simulink model "ThreeWheeledVehicle"  (R2017b)
settings: Solver=VariableStepAuto  StartTime=0.0  StopTime=25  RelTol=1e-3
undefined symbols (not defined in the file): b_contact_RW, C_F_alpha, C_F_kappa, CM_phi, Cylinder, Dtheta0, epsilon, g, k_contact_RW, lengthRW, massRW, Parts_Lib, radiusRW, sigbuilder_block, sigma, X, xPla, Y, yPla, Z, zPla
libraries: nesl_utility x42, sm_lib x39, vrlib x21, simulink x3
(part 2 of 3)

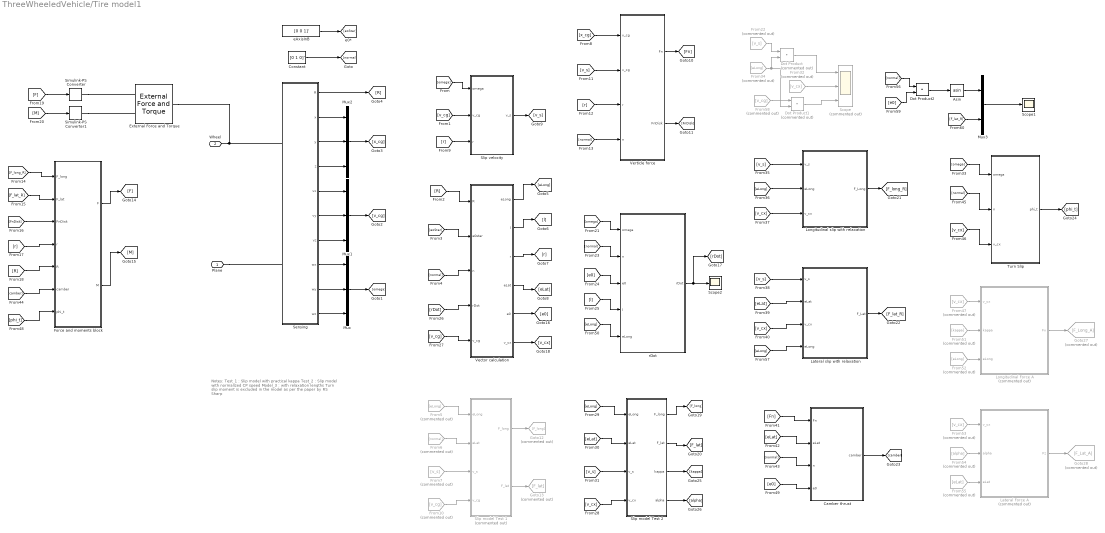
== system ThreeWheeledVehicle/Tire model1 ==
  note: Notes:
      | Test_1 : Slip model with practical kappa
      | Test_2 : Slip model with normalized CP speed
      | Model_3 : with relaxation lengths
      |
      | Turn slip moment is excluded in the model as per the
      | paper by RS Sharp
  Asin : Trigonometry  Operator=asin
  Camber thrust : Subsystem
  Constant : Constant  Value=[0 1 0]'
  Dot Product : DotProduct  Commented=on  InputSameDT=on  OutDataTypeStr=Inherit: Inherit via internal rule
  Dot Product1 : DotProduct  Commented=on  InputSameDT=on  OutDataTypeStr=Inherit: Inherit via internal rule
  Dot Product2 : DotProduct  InputSameDT=on  OutDataTypeStr=Inherit: Inherit via internal rule
  External Force and Torque : sm_lib/Forces and Torques/External Force and Torque  ForceResolutionFrame=AttachedFrame  EnableForceX=off  EnableForceY=off  EnableForceZ=off  EnableForce=on  TorqueResolutionFrame=AttachedFrame  EnableTorqueX=off  EnableTorqueY=off  EnableTorqueZ=off  EnableTorque=on
  Force and moments block : Subsystem
  From10 : From  Commented=on  GotoTag=v_cg
  From22 : From  Commented=on  GotoTag=v_s
  From32 : From  Commented=on  GotoTag=v_cx
  From34 : From  Commented=on  GotoTag=eLong
  From47 : From  Commented=on  GotoTag=v_cx
  From5 : From  Commented=on  GotoTag=eLong
  From51 : From  Commented=on  GotoTag=kappa
  From52 : From  Commented=on  GotoTag=eLong
  From53 : From  Commented=on  GotoTag=v_cx
  From54 : From  Commented=on  GotoTag=alpha
  From55 : From  Commented=on  GotoTag=eLat
  From58 : From  Commented=on  GotoTag=v_cg
  From6 : From  Commented=on  GotoTag=normal
  From7 : From  Commented=on  GotoTag=v_s
  Goto12 : Goto  Commented=on  GotoTag=F_long
  Goto13 : Goto  Commented=on  GotoTag=F_lat
  Goto27 : Goto  Commented=on  GotoTag=F_Long_A
  Goto28 : Goto  Commented=on  GotoTag=F_Lat_A
  Lateral Force A : Subsystem  Commented=on
  Lateral slip with relaxation : Subsystem
  Longitudinal Force A : Subsystem  Commented=on
  Longitudinal slip with relaxation : Subsystem
  Mux : Mux  Inputs=3
  Mux1 : Mux  Inputs=3
  Mux2 : Mux  Inputs=3
  Mux3 : Mux  Inputs=2
  Scope : Scope  Commented=on  NumInputPorts=3
  Scope1 : Scope
  Scope2 : Scope
  Sensing : Subsystem
  Simulink-PS Converter : nesl_utility/Simulink-PS Converter  PhysicalDomain=network_engine_domain  SubClassName=ps_input  LeftPortType=input  RightPortType=output  PseudoPeriodic=off  Frequencies=[]  NoiseDistribution=none  NoiseParameters=[]  Unit=N  AffineConversion=off  FilteringAndDerivatives=provide  SimscapeFilterOrder=1  InputFilterTimeConstant=0.001  UdotUserProvided=0
  Simulink-PS Converter1 : nesl_utility/Simulink-PS Converter  PhysicalDomain=network_engine_domain  SubClassName=ps_input  LeftPortType=input  RightPortType=output  PseudoPeriodic=off  Frequencies=[]  NoiseDistribution=none  NoiseParameters=[]  Unit=N*m  AffineConversion=off  FilteringAndDerivatives=provide  SimscapeFilterOrder=1  InputFilterTimeConstant=0.001  UdotUserProvided=0
  Slip model Test 1 : Subsystem  Commented=on
  Slip model Test 2 : Subsystem
  Slip velocity : Subsystem
  Turn Slip : Subsystem
  Vector calculation : Subsystem
  Verticle force : Subsystem
  eAxisInB : Constant  Value=[0 0 1]'
  rDot : Subsystem
  Plane : PMIOPort  Port=1  Side=Left
  Wheel : PMIOPort  Port=2  Side=Right
  wires:
  eAxisInB/1 -> [eoStar]
  Constant/1 -> [normal]
  Sensing/8(wx) -> Mux/1
  Sensing/9(wy) -> Mux/2
  Sensing/10(wz) -> Mux/3
  Mux/1 -> [omega]
  [omega] -> Slip velocity/1(omega)
  Sensing/5(vx) -> Mux1/1
  Sensing/6(vy) -> Mux1/2
  Sensing/7(vz) -> Mux1/3
  Mux1/1 -> [v_cg]
  [v_cg] -> Slip velocity/2(v_cg)
  Sensing/2(x) -> Mux2/1
  Sensing/3(y) -> Mux2/2
  Sensing/4(z) -> Mux2/3
  Mux2/1 -> [x_cg]
  Sensing/1(R) -> [R]
  [R] -> Vector calculation/1(R)
  [eoStar] -> Vector calculation/2(e0star)
  [normal] -> Vector calculation/3(n)
  From5/1 -> Slip model Test 1/1(eLong)
  From6/1 -> Slip model Test 1/2(eLat)
  Vector calculation/1(eLong) -> [eLong]
  Vector calculation/2(l) -> [l]
  Vector calculation/3(r) -> [r]
  Vector calculation/4(eLat) -> [eLat]
  [r] -> Slip velocity/3(r)
  Slip velocity/1(v_s) -> [v_s]
  From7/1 -> Slip model Test 1/3(v_s)
  From10/1 -> Slip model Test 1/4(v_cg)
  [x_cg] -> Verticle force/1(x_cg)
  [v_s] -> Verticle force/2(v_cg)
  [r] -> Verticle force/3(r)
  [normal] -> Verticle force/4(n)
  Verticle force/1(Fn) -> [Fn]
  Verticle force/2(FnDisk) -> [FnDisk]
  Slip model Test 1/1(F_long) -> Goto12/1
  Slip model Test 1/2(F_lat) -> Goto13/1
  [r] -> Force and moments block/4(r)
  [R] -> Force and moments block/5(R)
  [F] -> Simulink-PS Converter/1
  [M] -> Simulink-PS Converter1/1
  Vector calculation/5(e0) -> [e0]
  [v_cg] -> Vector calculation/5(v_cg)
  Vector calculation/6(v_cx) -> [v_cx]
  Slip model Test 2/1(F_long) -> [F_long]
  [v_s] -> Slip model Test 2/3(v_s)
  [eLat] -> Slip model Test 2/2(eLat)
  [eLong] -> Slip model Test 2/1(eLong)
  Slip model Test 2/2(F_lat) -> [F_lat]
  [v_cx] -> Slip model Test 2/4(v_cx)
  From22/1 -> Dot Product/1
  From34/1 -> Dot Product1/2, Dot Product/2
  Dot Product/1 -> Scope/1
  [v_s] -> Longitudinal slip with relaxation/1(v_s)
  [eLong] -> Longitudinal slip with relaxation/2(eLong)
  [v_cx] -> Longitudinal slip with relaxation/3(v_cx)
  Longitudinal slip with relaxation/1(F_Long) -> [F_long_R]
  [eLat] -> Lateral slip with relaxation/2(eLat)
  Lateral slip with relaxation/1(F_Lat) -> [F_lat_R]
  [v_cx] -> Lateral slip with relaxation/3(v_cx)
  [v_s] -> Lateral slip with relaxation/1(v_s)
  [Fn] -> Camber thrust/1(Fn)
  [eLat] -> Camber thrust/2(eLat)
  [normal] -> Camber thrust/3(n)
  Camber thrust/1(camber) -> [camber]
  [e0] -> Camber thrust/4(e0)
  Force and moments block/1(F) -> [F]
  Force and moments block/2(M) -> [M]
  [eLong] -> Lateral slip with relaxation/4(eLong)
  From32/1 -> Scope/2
  From58/1 -> Dot Product1/1
  Dot Product1/1 -> Scope/3
  [omega] -> rDot/1(omega)
  [normal] -> rDot/2(n)
  [e0] -> rDot/3(e0)
  [l] -> rDot/4(l)
  [eLong] -> rDot/5(eLong)
  rDot/1(rDot) -> [rDot], Scope2/1
  [rDot] -> Vector calculation/4(rDot)
  Slip model Test 2/3(kappa) -> [kappa]
  [omega] -> Turn Slip/1(omega)
  [normal] -> Turn Slip/2(n)
  [v_cx] -> Turn Slip/3(v_cx)
  Turn Slip/1(phi_t) -> [phi_t]
  From47/1 -> Longitudinal Force A/1(v_cx)
  Slip model Test 2/4(alpha) -> [alpha]
  From51/1 -> Longitudinal Force A/2(kappa)
  From52/1 -> Longitudinal Force A/3(eLong)
  Longitudinal Force A/1(Fx) -> Goto27/1
  From53/1 -> Lateral Force A/1(v_cx)
  From54/1 -> Lateral Force A/2(alpha)
  From55/1 -> Lateral Force A/3(eLat)
  Lateral Force A/1(Fz) -> Goto28/1
  [normal] -> Dot Product2/1
  [e0] -> Dot Product2/2
  Dot Product2/1 -> Asin/1
  Asin/1 -> Mux3/1
  [F_lat_R] -> Mux3/2
  Mux3/1 -> Scope1/1
  [FnDisk] -> Force and moments block/3(FnDisk)
  [F_long_R] -> Force and moments block/1(F_long)
  [F_lat_R] -> Force and moments block/2(F_lat)
  [camber] -> Force and moments block/6(camber)
  [phi_t] -> Force and moments block/7(phi_t)
  connections:
  Plane/RConn1 -- Sensing/LConn2
  Wheel/RConn1 -- External Force and Torque/RConn1 -- Sensing/LConn1
  Simulink-PS Converter/RConn1 -- External Force and Torque/LConn1
  Simulink-PS Converter1/RConn1 -- External Force and Torque/LConn2

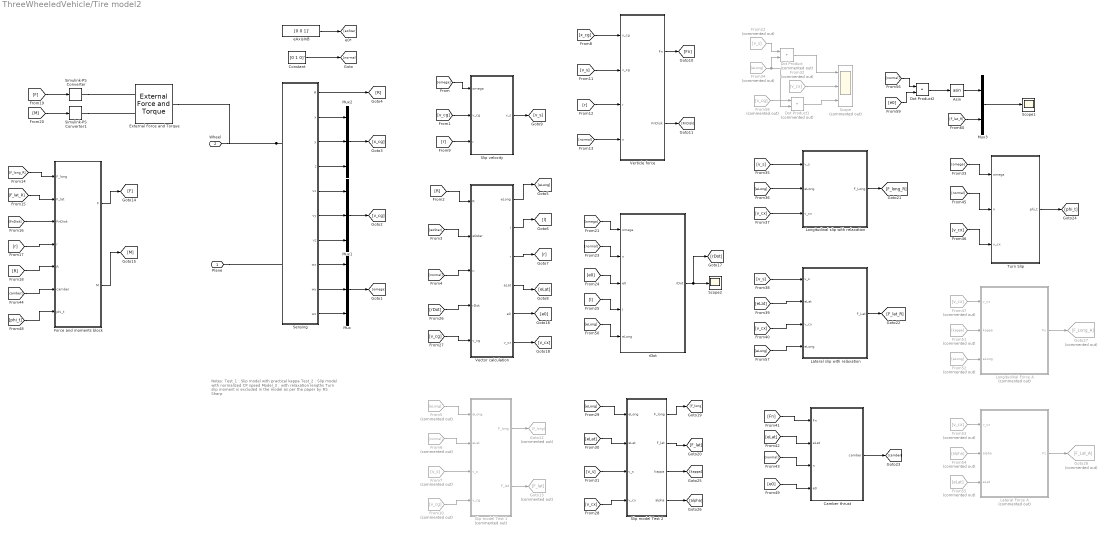
== system ThreeWheeledVehicle/Tire model2 ==
  note: Notes:
      | Test_1 : Slip model with practical kappa
      | Test_2 : Slip model with normalized CP speed
      | Model_3 : with relaxation lengths
      |
      | Turn slip moment is excluded in the model as per the
      | paper by RS Sharp
  Asin : Trigonometry  Operator=asin
  Camber thrust : Subsystem
  Constant : Constant  Value=[0 1 0]'
  Dot Product : DotProduct  Commented=on  InputSameDT=on  OutDataTypeStr=Inherit: Inherit via internal rule
  Dot Product1 : DotProduct  Commented=on  InputSameDT=on  OutDataTypeStr=Inherit: Inherit via internal rule
  Dot Product2 : DotProduct  InputSameDT=on  OutDataTypeStr=Inherit: Inherit via internal rule
  External Force and Torque : sm_lib/Forces and Torques/External Force and Torque  ForceResolutionFrame=AttachedFrame  EnableForceX=off  EnableForceY=off  EnableForceZ=off  EnableForce=on  TorqueResolutionFrame=AttachedFrame  EnableTorqueX=off  EnableTorqueY=off  EnableTorqueZ=off  EnableTorque=on
  Force and moments block : Subsystem
  From10 : From  Commented=on  GotoTag=v_cg
  From22 : From  Commented=on  GotoTag=v_s
  From32 : From  Commented=on  GotoTag=v_cx
  From34 : From  Commented=on  GotoTag=eLong
  From47 : From  Commented=on  GotoTag=v_cx
  From5 : From  Commented=on  GotoTag=eLong
  From51 : From  Commented=on  GotoTag=kappa
  From52 : From  Commented=on  GotoTag=eLong
  From53 : From  Commented=on  GotoTag=v_cx
  From54 : From  Commented=on  GotoTag=alpha
  From55 : From  Commented=on  GotoTag=eLat
  From58 : From  Commented=on  GotoTag=v_cg
  From6 : From  Commented=on  GotoTag=normal
  From7 : From  Commented=on  GotoTag=v_s
  Goto12 : Goto  Commented=on  GotoTag=F_long
  Goto13 : Goto  Commented=on  GotoTag=F_lat
  Goto27 : Goto  Commented=on  GotoTag=F_Long_A
  Goto28 : Goto  Commented=on  GotoTag=F_Lat_A
  Lateral Force A : Subsystem  Commented=on
  Lateral slip with relaxation : Subsystem
  Longitudinal Force A : Subsystem  Commented=on
  Longitudinal slip with relaxation : Subsystem
  Mux : Mux  Inputs=3
  Mux1 : Mux  Inputs=3
  Mux2 : Mux  Inputs=3
  Mux3 : Mux  Inputs=2
  Scope : Scope  Commented=on  NumInputPorts=3
  Scope1 : Scope
  Scope2 : Scope
  Sensing : Subsystem
  Simulink-PS Converter : nesl_utility/Simulink-PS Converter  PhysicalDomain=network_engine_domain  SubClassName=ps_input  LeftPortType=input  RightPortType=output  PseudoPeriodic=off  Frequencies=[]  NoiseDistribution=none  NoiseParameters=[]  Unit=N  AffineConversion=off  FilteringAndDerivatives=provide  SimscapeFilterOrder=1  InputFilterTimeConstant=0.001  UdotUserProvided=0
  Simulink-PS Converter1 : nesl_utility/Simulink-PS Converter  PhysicalDomain=network_engine_domain  SubClassName=ps_input  LeftPortType=input  RightPortType=output  PseudoPeriodic=off  Frequencies=[]  NoiseDistribution=none  NoiseParameters=[]  Unit=N*m  AffineConversion=off  FilteringAndDerivatives=provide  SimscapeFilterOrder=1  InputFilterTimeConstant=0.001  UdotUserProvided=0
  Slip model Test 1 : Subsystem  Commented=on
  Slip model Test 2 : Subsystem
  Slip velocity : Subsystem
  Turn Slip : Subsystem
  Vector calculation : Subsystem
  Verticle force : Subsystem
  eAxisInB : Constant  Value=[0 0 1]'
  rDot : Subsystem
  Plane : PMIOPort  Port=1  Side=Left
  Wheel : PMIOPort  Port=2  Side=Right
  wires:
  [camber] -> Force and moments block/6(camber)
  [F_lat_R] -> Force and moments block/2(F_lat)
  [F_long_R] -> Force and moments block/1(F_long)
  [FnDisk] -> Force and moments block/3(FnDisk)
  Mux3/1 -> Scope1/1
  [F_lat_R] -> Mux3/2
  Asin/1 -> Mux3/1
  Dot Product2/1 -> Asin/1
  [e0] -> Dot Product2/2
  [normal] -> Dot Product2/1
  Lateral Force A/1(Fz) -> Goto28/1
  From55/1 -> Lateral Force A/3(eLat)
  From54/1 -> Lateral Force A/2(alpha)
  From53/1 -> Lateral Force A/1(v_cx)
  Longitudinal Force A/1(Fx) -> Goto27/1
  From52/1 -> Longitudinal Force A/3(eLong)
  From51/1 -> Longitudinal Force A/2(kappa)
  Slip model Test 2/4(alpha) -> [alpha]
  From47/1 -> Longitudinal Force A/1(v_cx)
  Turn Slip/1(phi_t) -> [phi_t]
  [v_cx] -> Turn Slip/3(v_cx)
  [normal] -> Turn Slip/2(n)
  [omega] -> Turn Slip/1(omega)
  Slip model Test 2/3(kappa) -> [kappa]
  [rDot] -> Vector calculation/4(rDot)
  rDot/1(rDot) -> Scope2/1, [rDot]
  [eLong] -> rDot/5(eLong)
  [l] -> rDot/4(l)
  [e0] -> rDot/3(e0)
  [normal] -> rDot/2(n)
  [omega] -> rDot/1(omega)
  Dot Product1/1 -> Scope/3
  From58/1 -> Dot Product1/1
  From32/1 -> Scope/2
  [eLong] -> Lateral slip with relaxation/4(eLong)
  Force and moments block/2(M) -> [M]
  Force and moments block/1(F) -> [F]
  [e0] -> Camber thrust/4(e0)
  Camber thrust/1(camber) -> [camber]
  [normal] -> Camber thrust/3(n)
  [eLat] -> Camber thrust/2(eLat)
  [Fn] -> Camber thrust/1(Fn)
  [v_s] -> Lateral slip with relaxation/1(v_s)
  [v_cx] -> Lateral slip with relaxation/3(v_cx)
  Lateral slip with relaxation/1(F_Lat) -> [F_lat_R]
  [eLat] -> Lateral slip with relaxation/2(eLat)
  Longitudinal slip with relaxation/1(F_Long) -> [F_long_R]
  [v_cx] -> Longitudinal slip with relaxation/3(v_cx)
  [eLong] -> Longitudinal slip with relaxation/2(eLong)
  [v_s] -> Longitudinal slip with relaxation/1(v_s)
  Dot Product/1 -> Scope/1
  From34/1 -> Dot Product/2, Dot Product1/2
  From22/1 -> Dot Product/1
  [v_cx] -> Slip model Test 2/4(v_cx)
  Slip model Test 2/2(F_lat) -> [F_lat]
  [eLong] -> Slip model Test 2/1(eLong)
  [eLat] -> Slip model Test 2/2(eLat)
  [v_s] -> Slip model Test 2/3(v_s)
  Slip model Test 2/1(F_long) -> [F_long]
  Vector calculation/6(v_cx) -> [v_cx]
  [v_cg] -> Vector calculation/5(v_cg)
  Vector calculation/5(e0) -> [e0]
  [M] -> Simulink-PS Converter1/1
  [F] -> Simulink-PS Converter/1
  [R] -> Force and moments block/5(R)
  [r] -> Force and moments block/4(r)
  Slip model Test 1/2(F_lat) -> Goto13/1
  Slip model Test 1/1(F_long) -> Goto12/1
  Verticle force/2(FnDisk) -> [FnDisk]
  Verticle force/1(Fn) -> [Fn]
  [normal] -> Verticle force/4(n)
  [r] -> Verticle force/3(r)
  [v_s] -> Verticle force/2(v_cg)
  [x_cg] -> Verticle force/1(x_cg)
  From10/1 -> Slip model Test 1/4(v_cg)
  From7/1 -> Slip model Test 1/3(v_s)
  Slip velocity/1(v_s) -> [v_s]
  [r] -> Slip velocity/3(r)
  Vector calculation/4(eLat) -> [eLat]
  Vector calculation/3(r) -> [r]
  Vector calculation/2(l) -> [l]
  Vector calculation/1(eLong) -> [eLong]
  From6/1 -> Slip model Test 1/2(eLat)
  From5/1 -> Slip model Test 1/1(eLong)
  [normal] -> Vector calculation/3(n)
  [eoStar] -> Vector calculation/2(e0star)
  [R] -> Vector calculation/1(R)
  Sensing/1(R) -> [R]
  Mux2/1 -> [x_cg]
  Sensing/4(z) -> Mux2/3
  Sensing/3(y) -> Mux2/2
  Sensing/2(x) -> Mux2/1
  [v_cg] -> Slip velocity/2(v_cg)
  Mux1/1 -> [v_cg]
  Sensing/7(vz) -> Mux1/3
  Sensing/6(vy) -> Mux1/2
  Sensing/5(vx) -> Mux1/1
  [omega] -> Slip velocity/1(omega)
  Mux/1 -> [omega]
  Sensing/10(wz) -> Mux/3
  Sensing/9(wy) -> Mux/2
  Sensing/8(wx) -> Mux/1
  Constant/1 -> [normal]
  eAxisInB/1 -> [eoStar]
  [phi_t] -> Force and moments block/7(phi_t)
  connections:
  Simulink-PS Converter1/RConn1 -- External Force and Torque/LConn2
  Simulink-PS Converter/RConn1 -- External Force and Torque/LConn1
  Sensing/LConn1 -- External Force and Torque/RConn1 -- Wheel/RConn1
  Plane/RConn1 -- Sensing/LConn2

== system ThreeWheeledVehicle/Wheel_Front ==
  Cylinder : sm_lib/Body Elements/Solid  InertiaType=Custom  Mass=massRW  MassUnits=kg  CenterOfMass=[0 0 0]  CenterOfMassUnits=m  MomentsOfInertia=momentInertiaRW  MomentsOfInertiaUnits=kg*m^2  ProductsOfInertia=[0 0 0]  ProductsOfInertiaUnits=kg*m^2  DensityBased=on  Density=cyl_density  DensityUnits=kg/(m^3)  DoExposeReferenceFrame=on  SerializedFrames=<Frames/>  GraphicType=FromGeometry  MarkerShape=Sphere  MarkerSize=10  MarkerSizeUnits=m  GraphicVisPropType=SimpleVisualProperties  GraphicDiffuseColor=[0.0 0.5 0.7]  GraphicSpecularColor=[0.5 0.5 0.5 1.0]  GraphicAmbientColor=[0.15 0.15 0.15 1.0]  GraphicEmissiveColor=[0.0 0.0 0.0 1.0]  GraphicShininess=75  GraphicOpacity=cyl_opacity  GeometryShape=Cylinder  RectangleSize=[1 1]  RectangleSizeUnits=m  BrickDimensions=[1 1 1]  BrickDimensionUnits=m  CylinderRadius=cyl_radius  CylinderRadiusUnits=m  CylinderLength=cyl_length  CylinderLengthUnits=m  SphereRadius=1  SphereRadiusUnits=m  EllipsoidRadii=[1 1 1]  EllipsoidRadiiUnits=m  ExtrusionCrossSection=[1 1; -1 1; -1 -1; 1 -1]  ExtrusionCrossSectionUnits=m  ExtrusionLength=1  ExtrusionLengthUnits=m  PolygonNumSides=3  PolygonOuterRadius=1  PolygonOuterRadiusUnits=m  ExtGeomFileType=STL  ExtGeomFileUnits=m  RevolutionCrossSection=[1 1; 1 -1; 2 -1; 2 1]  RevolutionCrossSectionUnits=m  RevolutionExtent=Full  RevolutionAngle=180  RevolutionAngleUnits=deg
  Transform Vis2 : sm_lib/Frames and Transforms/Rigid Transform  TranslationMethod=None  TranslationStandardOffset=0  TranslationLengthUnit=m  TranslationStandardAxis=+Z  TranslationCartesianOffset=[0 0 0]  TranslationROffset=0  TranslationROffsetUnits=m  TranslationZOffset=0  TranslationZOffsetUnits=m  TranslationThetaOffset=0  TranslationThetaOffsetUnits=deg  RotationMethod=StandardAxis  RotationAngleUnits=deg  RotationStandardAxis=+Y  RotationAngle=180  RotationArbitraryAxis=[0 0 1]  FollAlignAxisA=+X  BaseAlignAxisA=+Y  FollAlignAxisB=+Y  BaseAlignAxisB=+Z  RotationSequenceAxes=FollowerAxes  RotationSequence=XYX  RotationSequenceAngles=[0 0 0]  RotationSequenceAnglesUnits=deg  RotationMatrix=[1 0 0; 0 1 0; 0 0 1]
  Vis1 : sm_lib/Body Elements/Solid  InertiaType=CalculateFromGeometry  Mass=1  MassUnits=kg  CenterOfMass=[0 0 0]  CenterOfMassUnits=m  MomentsOfInertia=[1 1 1]  MomentsOfInertiaUnits=kg*m^2  ProductsOfInertia=[0 0 0]  ProductsOfInertiaUnits=kg*m^2  DensityBased=on  Density=1e-3  DensityUnits=kg/(m^3)  DoExposeReferenceFrame=on  SerializedFrames=<Frames/>  GraphicType=FromGeometry  MarkerShape=Sphere  MarkerSize=10  MarkerSizeUnits=m  GraphicVisPropType=SimpleVisualProperties  GraphicDiffuseColor=[0.4 0.0 0.4]  GraphicSpecularColor=[0.5 0.5 0.5 1.0]  GraphicAmbientColor=[0.15 0.15 0.15 1.0]  GraphicEmissiveColor=[0.0 0.0 0.0 1.0]  GraphicShininess=75  GraphicOpacity=mark_opacity  GeometryShape=GeneralSolidOfRevolution  RectangleSize=[1 1]  RectangleSizeUnits=m  BrickDimensions=[1 1 1]  BrickDimensionUnits=m  CylinderRadius=0.1  CylinderRadiusUnits=m  CylinderLength=0.01  CylinderLengthUnits=m  SphereRadius=1  SphereRadiusUnits=m  EllipsoidRadii=[1 1 1]  EllipsoidRadiiUnits=m  ExtrusionCrossSection=[1 1; -1 1; -1 -1; 1 -1]  ExtrusionCrossSectionUnits=m  ExtrusionLength=1  ExtrusionLengthUnits=m  PolygonNumSides=3  PolygonOuterRadius=1  PolygonOuterRadiusUnits=m  ExtGeomFileType=STL  ExtGeomFileUnits=m  RevolutionCrossSection=[cyl_radius*mark_radius(1) cyl_length/2*mark_len_factor; cyl_radius*mark_radius(2) cyl_length/2*mark_len_factor; cyl_radius*mark_radius(2) -cyl_length/2*mark_len_factor; cyl_radius*mark_radius(1) -cyl_length/2*mark_len_factor]  RevolutionCrossSectionUnits=m  RevolutionExtent=Custom  RevolutionAngle=mark_angle  RevolutionAngleUnits=deg
  Vis2 : sm_lib/Body Elements/Solid  InertiaType=CalculateFromGeometry  Mass=1  MassUnits=kg  CenterOfMass=[0 0 0]  CenterOfMassUnits=m  MomentsOfInertia=[1 1 1]  MomentsOfInertiaUnits=kg*m^2  ProductsOfInertia=[0 0 0]  ProductsOfInertiaUnits=kg*m^2  DensityBased=on  Density=1e-3  DensityUnits=kg/(m^3)  DoExposeReferenceFrame=on  SerializedFrames=<Frames/>  GraphicType=FromGeometry  MarkerShape=Sphere  MarkerSize=10  MarkerSizeUnits=m  GraphicVisPropType=SimpleVisualProperties  GraphicDiffuseColor=[0.4 0.0 0.4]  GraphicSpecularColor=[0.5 0.5 0.5 1.0]  GraphicAmbientColor=[0.15 0.15 0.15 1.0]  GraphicEmissiveColor=[0.0 0.0 0.0 1.0]  GraphicShininess=75  GraphicOpacity=mark_opacity  GeometryShape=GeneralSolidOfRevolution  RectangleSize=[1 1]  RectangleSizeUnits=m  BrickDimensions=[1 1 1]  BrickDimensionUnits=m  CylinderRadius=0.1  CylinderRadiusUnits=m  CylinderLength=0.01  CylinderLengthUnits=m  SphereRadius=1  SphereRadiusUnits=m  EllipsoidRadii=[1 1 1]  EllipsoidRadiiUnits=m  ExtrusionCrossSection=[1 1; -1 1; -1 -1; 1 -1]  ExtrusionCrossSectionUnits=m  ExtrusionLength=1  ExtrusionLengthUnits=m  PolygonNumSides=3  PolygonOuterRadius=1  PolygonOuterRadiusUnits=m  ExtGeomFileType=STL  ExtGeomFileUnits=m  RevolutionCrossSection=[cyl_radius*mark_radius(1) cyl_length/2*mark_len_factor; cyl_radius*mark_radius(2) cyl_length/2*mark_len_factor; cyl_radius*mark_radius(2) -cyl_length/2*mark_len_factor; cyl_radius*mark_radius(1) -cyl_length/2*mark_len_factor]  RevolutionCrossSectionUnits=m  RevolutionExtent=Custom  RevolutionAngle=mark_angle  RevolutionAngleUnits=deg
  R : PMIOPort  Port=1  Side=Left
  connections:
  R/RConn1 -- Cylinder/RConn1 -- Transform Vis2/LConn1 -- Vis1/RConn1
  Vis2/RConn1 -- Transform Vis2/RConn1

== system ThreeWheeledVehicle/Wheel_RW_L ==
  Cylinder : sm_lib/Body Elements/Solid  InertiaType=Custom  Mass=massRW  MassUnits=kg  CenterOfMass=[0 0 0]  CenterOfMassUnits=m  MomentsOfInertia=momentInertiaRW  MomentsOfInertiaUnits=kg*m^2  ProductsOfInertia=[0 0 0]  ProductsOfInertiaUnits=kg*m^2  DensityBased=on  Density=cyl_density  DensityUnits=kg/(m^3)  DoExposeReferenceFrame=on  SerializedFrames=<Frames/>  GraphicType=FromGeometry  MarkerShape=Sphere  MarkerSize=10  MarkerSizeUnits=m  GraphicVisPropType=SimpleVisualProperties  GraphicDiffuseColor=[0.0 0.5 0.7]  GraphicSpecularColor=[0.5 0.5 0.5 1.0]  GraphicAmbientColor=[0.15 0.15 0.15 1.0]  GraphicEmissiveColor=[0.0 0.0 0.0 1.0]  GraphicShininess=75  GraphicOpacity=cyl_opacity  GeometryShape=Cylinder  RectangleSize=[1 1]  RectangleSizeUnits=m  BrickDimensions=[1 1 1]  BrickDimensionUnits=m  CylinderRadius=cyl_radius  CylinderRadiusUnits=m  CylinderLength=cyl_length  CylinderLengthUnits=m  SphereRadius=1  SphereRadiusUnits=m  EllipsoidRadii=[1 1 1]  EllipsoidRadiiUnits=m  ExtrusionCrossSection=[1 1; -1 1; -1 -1; 1 -1]  ExtrusionCrossSectionUnits=m  ExtrusionLength=1  ExtrusionLengthUnits=m  PolygonNumSides=3  PolygonOuterRadius=1  PolygonOuterRadiusUnits=m  ExtGeomFileType=STL  ExtGeomFileUnits=m  RevolutionCrossSection=[1 1; 1 -1; 2 -1; 2 1]  RevolutionCrossSectionUnits=m  RevolutionExtent=Full  RevolutionAngle=180  RevolutionAngleUnits=deg
  Transform Vis2 : sm_lib/Frames and Transforms/Rigid Transform  TranslationMethod=None  TranslationStandardOffset=0  TranslationLengthUnit=m  TranslationStandardAxis=+Z  TranslationCartesianOffset=[0 0 0]  TranslationROffset=0  TranslationROffsetUnits=m  TranslationZOffset=0  TranslationZOffsetUnits=m  TranslationThetaOffset=0  TranslationThetaOffsetUnits=deg  RotationMethod=StandardAxis  RotationAngleUnits=deg  RotationStandardAxis=+Y  RotationAngle=180  RotationArbitraryAxis=[0 0 1]  FollAlignAxisA=+X  BaseAlignAxisA=+Y  FollAlignAxisB=+Y  BaseAlignAxisB=+Z  RotationSequenceAxes=FollowerAxes  RotationSequence=XYX  RotationSequenceAngles=[0 0 0]  RotationSequenceAnglesUnits=deg  RotationMatrix=[1 0 0; 0 1 0; 0 0 1]
  Vis1 : sm_lib/Body Elements/Solid  InertiaType=CalculateFromGeometry  Mass=1  MassUnits=kg  CenterOfMass=[0 0 0]  CenterOfMassUnits=m  MomentsOfInertia=[1 1 1]  MomentsOfInertiaUnits=kg*m^2  ProductsOfInertia=[0 0 0]  ProductsOfInertiaUnits=kg*m^2  DensityBased=on  Density=1e-3  DensityUnits=kg/(m^3)  DoExposeReferenceFrame=on  SerializedFrames=<Frames/>  GraphicType=FromGeometry  MarkerShape=Sphere  MarkerSize=10  MarkerSizeUnits=m  GraphicVisPropType=SimpleVisualProperties  GraphicDiffuseColor=[0.4 0.0 0.4]  GraphicSpecularColor=[0.5 0.5 0.5 1.0]  GraphicAmbientColor=[0.15 0.15 0.15 1.0]  GraphicEmissiveColor=[0.0 0.0 0.0 1.0]  GraphicShininess=75  GraphicOpacity=mark_opacity  GeometryShape=GeneralSolidOfRevolution  RectangleSize=[1 1]  RectangleSizeUnits=m  BrickDimensions=[1 1 1]  BrickDimensionUnits=m  CylinderRadius=0.1  CylinderRadiusUnits=m  CylinderLength=0.01  CylinderLengthUnits=m  SphereRadius=1  SphereRadiusUnits=m  EllipsoidRadii=[1 1 1]  EllipsoidRadiiUnits=m  ExtrusionCrossSection=[1 1; -1 1; -1 -1; 1 -1]  ExtrusionCrossSectionUnits=m  ExtrusionLength=1  ExtrusionLengthUnits=m  PolygonNumSides=3  PolygonOuterRadius=1  PolygonOuterRadiusUnits=m  ExtGeomFileType=STL  ExtGeomFileUnits=m  RevolutionCrossSection=[cyl_radius*mark_radius(1) cyl_length/2*mark_len_factor; cyl_radius*mark_radius(2) cyl_length/2*mark_len_factor; cyl_radius*mark_radius(2) -cyl_length/2*mark_len_factor; cyl_radius*mark_radius(1) -cyl_length/2*mark_len_factor]  RevolutionCrossSectionUnits=m  RevolutionExtent=Custom  RevolutionAngle=mark_angle  RevolutionAngleUnits=deg
  Vis2 : sm_lib/Body Elements/Solid  InertiaType=CalculateFromGeometry  Mass=1  MassUnits=kg  CenterOfMass=[0 0 0]  CenterOfMassUnits=m  MomentsOfInertia=[1 1 1]  MomentsOfInertiaUnits=kg*m^2  ProductsOfInertia=[0 0 0]  ProductsOfInertiaUnits=kg*m^2  DensityBased=on  Density=1e-3  DensityUnits=kg/(m^3)  DoExposeReferenceFrame=on  SerializedFrames=<Frames/>  GraphicType=FromGeometry  MarkerShape=Sphere  MarkerSize=10  MarkerSizeUnits=m  GraphicVisPropType=SimpleVisualProperties  GraphicDiffuseColor=[0.4 0.0 0.4]  GraphicSpecularColor=[0.5 0.5 0.5 1.0]  GraphicAmbientColor=[0.15 0.15 0.15 1.0]  GraphicEmissiveColor=[0.0 0.0 0.0 1.0]  GraphicShininess=75  GraphicOpacity=mark_opacity  GeometryShape=GeneralSolidOfRevolution  RectangleSize=[1 1]  RectangleSizeUnits=m  BrickDimensions=[1 1 1]  BrickDimensionUnits=m  CylinderRadius=0.1  CylinderRadiusUnits=m  CylinderLength=0.01  CylinderLengthUnits=m  SphereRadius=1  SphereRadiusUnits=m  EllipsoidRadii=[1 1 1]  EllipsoidRadiiUnits=m  ExtrusionCrossSection=[1 1; -1 1; -1 -1; 1 -1]  ExtrusionCrossSectionUnits=m  ExtrusionLength=1  ExtrusionLengthUnits=m  PolygonNumSides=3  PolygonOuterRadius=1  PolygonOuterRadiusUnits=m  ExtGeomFileType=STL  ExtGeomFileUnits=m  RevolutionCrossSection=[cyl_radius*mark_radius(1) cyl_length/2*mark_len_factor; cyl_radius*mark_radius(2) cyl_length/2*mark_len_factor; cyl_radius*mark_radius(2) -cyl_length/2*mark_len_factor; cyl_radius*mark_radius(1) -cyl_length/2*mark_len_factor]  RevolutionCrossSectionUnits=m  RevolutionExtent=Custom  RevolutionAngle=mark_angle  RevolutionAngleUnits=deg
  R : PMIOPort  Port=1  Side=Left
  connections:
  Vis2/RConn1 -- Transform Vis2/RConn1
  Vis1/RConn1 -- Transform Vis2/LConn1 -- Cylinder/RConn1 -- R/RConn1

== system ThreeWheeledVehicle/Wheel_RW_R ==
  Cylinder : sm_lib/Body Elements/Solid  InertiaType=Custom  Mass=massRW  MassUnits=kg  CenterOfMass=[0 0 0]  CenterOfMassUnits=m  MomentsOfInertia=momentInertiaRW  MomentsOfInertiaUnits=kg*m^2  ProductsOfInertia=[0 0 0]  ProductsOfInertiaUnits=kg*m^2  DensityBased=on  Density=cyl_density  DensityUnits=kg/(m^3)  DoExposeReferenceFrame=on  SerializedFrames=<Frames/>  GraphicType=FromGeometry  MarkerShape=Sphere  MarkerSize=10  MarkerSizeUnits=m  GraphicVisPropType=SimpleVisualProperties  GraphicDiffuseColor=[0.0 0.5 0.7]  GraphicSpecularColor=[0.5 0.5 0.5 1.0]  GraphicAmbientColor=[0.15 0.15 0.15 1.0]  GraphicEmissiveColor=[0.0 0.0 0.0 1.0]  GraphicShininess=75  GraphicOpacity=cyl_opacity  GeometryShape=Cylinder  RectangleSize=[1 1]  RectangleSizeUnits=m  BrickDimensions=[1 1 1]  BrickDimensionUnits=m  CylinderRadius=cyl_radius  CylinderRadiusUnits=m  CylinderLength=cyl_length  CylinderLengthUnits=m  SphereRadius=1  SphereRadiusUnits=m  EllipsoidRadii=[1 1 1]  EllipsoidRadiiUnits=m  ExtrusionCrossSection=[1 1; -1 1; -1 -1; 1 -1]  ExtrusionCrossSectionUnits=m  ExtrusionLength=1  ExtrusionLengthUnits=m  PolygonNumSides=3  PolygonOuterRadius=1  PolygonOuterRadiusUnits=m  ExtGeomFileType=STL  ExtGeomFileUnits=m  RevolutionCrossSection=[1 1; 1 -1; 2 -1; 2 1]  RevolutionCrossSectionUnits=m  RevolutionExtent=Full  RevolutionAngle=180  RevolutionAngleUnits=deg
  Transform Vis2 : sm_lib/Frames and Transforms/Rigid Transform  TranslationMethod=None  TranslationStandardOffset=0  TranslationLengthUnit=m  TranslationStandardAxis=+Z  TranslationCartesianOffset=[0 0 0]  TranslationROffset=0  TranslationROffsetUnits=m  TranslationZOffset=0  TranslationZOffsetUnits=m  TranslationThetaOffset=0  TranslationThetaOffsetUnits=deg  RotationMethod=StandardAxis  RotationAngleUnits=deg  RotationStandardAxis=+Y  RotationAngle=180  RotationArbitraryAxis=[0 0 1]  FollAlignAxisA=+X  BaseAlignAxisA=+Y  FollAlignAxisB=+Y  BaseAlignAxisB=+Z  RotationSequenceAxes=FollowerAxes  RotationSequence=XYX  RotationSequenceAngles=[0 0 0]  RotationSequenceAnglesUnits=deg  RotationMatrix=[1 0 0; 0 1 0; 0 0 1]
  Vis1 : sm_lib/Body Elements/Solid  InertiaType=CalculateFromGeometry  Mass=1  MassUnits=kg  CenterOfMass=[0 0 0]  CenterOfMassUnits=m  MomentsOfInertia=[1 1 1]  MomentsOfInertiaUnits=kg*m^2  ProductsOfInertia=[0 0 0]  ProductsOfInertiaUnits=kg*m^2  DensityBased=on  Density=1e-3  DensityUnits=kg/(m^3)  DoExposeReferenceFrame=on  SerializedFrames=<Frames/>  GraphicType=FromGeometry  MarkerShape=Sphere  MarkerSize=10  MarkerSizeUnits=m  GraphicVisPropType=SimpleVisualProperties  GraphicDiffuseColor=[0.4 0.0 0.4]  GraphicSpecularColor=[0.5 0.5 0.5 1.0]  GraphicAmbientColor=[0.15 0.15 0.15 1.0]  GraphicEmissiveColor=[0.0 0.0 0.0 1.0]  GraphicShininess=75  GraphicOpacity=mark_opacity  GeometryShape=GeneralSolidOfRevolution  RectangleSize=[1 1]  RectangleSizeUnits=m  BrickDimensions=[1 1 1]  BrickDimensionUnits=m  CylinderRadius=0.1  CylinderRadiusUnits=m  CylinderLength=0.01  CylinderLengthUnits=m  SphereRadius=1  SphereRadiusUnits=m  EllipsoidRadii=[1 1 1]  EllipsoidRadiiUnits=m  ExtrusionCrossSection=[1 1; -1 1; -1 -1; 1 -1]  ExtrusionCrossSectionUnits=m  ExtrusionLength=1  ExtrusionLengthUnits=m  PolygonNumSides=3  PolygonOuterRadius=1  PolygonOuterRadiusUnits=m  ExtGeomFileType=STL  ExtGeomFileUnits=m  RevolutionCrossSection=[cyl_radius*mark_radius(1) cyl_length/2*mark_len_factor; cyl_radius*mark_radius(2) cyl_length/2*mark_len_factor; cyl_radius*mark_radius(2) -cyl_length/2*mark_len_factor; cyl_radius*mark_radius(1) -cyl_length/2*mark_len_factor]  RevolutionCrossSectionUnits=m  RevolutionExtent=Custom  RevolutionAngle=mark_angle  RevolutionAngleUnits=deg
  Vis2 : sm_lib/Body Elements/Solid  InertiaType=CalculateFromGeometry  Mass=1  MassUnits=kg  CenterOfMass=[0 0 0]  CenterOfMassUnits=m  MomentsOfInertia=[1 1 1]  MomentsOfInertiaUnits=kg*m^2  ProductsOfInertia=[0 0 0]  ProductsOfInertiaUnits=kg*m^2  DensityBased=on  Density=1e-3  DensityUnits=kg/(m^3)  DoExposeReferenceFrame=on  SerializedFrames=<Frames/>  GraphicType=FromGeometry  MarkerShape=Sphere  MarkerSize=10  MarkerSizeUnits=m  GraphicVisPropType=SimpleVisualProperties  GraphicDiffuseColor=[0.4 0.0 0.4]  GraphicSpecularColor=[0.5 0.5 0.5 1.0]  GraphicAmbientColor=[0.15 0.15 0.15 1.0]  GraphicEmissiveColor=[0.0 0.0 0.0 1.0]  GraphicShininess=75  GraphicOpacity=mark_opacity  GeometryShape=GeneralSolidOfRevolution  RectangleSize=[1 1]  RectangleSizeUnits=m  BrickDimensions=[1 1 1]  BrickDimensionUnits=m  CylinderRadius=0.1  CylinderRadiusUnits=m  CylinderLength=0.01  CylinderLengthUnits=m  SphereRadius=1  SphereRadiusUnits=m  EllipsoidRadii=[1 1 1]  EllipsoidRadiiUnits=m  ExtrusionCrossSection=[1 1; -1 1; -1 -1; 1 -1]  ExtrusionCrossSectionUnits=m  ExtrusionLength=1  ExtrusionLengthUnits=m  PolygonNumSides=3  PolygonOuterRadius=1  PolygonOuterRadiusUnits=m  ExtGeomFileType=STL  ExtGeomFileUnits=m  RevolutionCrossSection=[cyl_radius*mark_radius(1) cyl_length/2*mark_len_factor; cyl_radius*mark_radius(2) cyl_length/2*mark_len_factor; cyl_radius*mark_radius(2) -cyl_length/2*mark_len_factor; cyl_radius*mark_radius(1) -cyl_length/2*mark_len_factor]  RevolutionCrossSectionUnits=m  RevolutionExtent=Custom  RevolutionAngle=mark_angle  RevolutionAngleUnits=deg
  R : PMIOPort  Port=1  Side=Left
  connections:
  Vis2/RConn1 -- Transform Vis2/RConn1
  Vis1/RConn1 -- Transform Vis2/LConn1 -- Cylinder/RConn1 -- R/RConn1

== system ThreeWheeledVehicle/Tire model/Camber thrust ==
  Fn : Inport
  eLat : Inport  Port=2
  n : Inport  Port=3
  e0 : Inport  Port=4
  Compare To Constant : simulink/Logic and Bit Operations/Compare To Constant  relop=<=  const=-1  OutDataTypeStr=boolean
  Dot Product : DotProduct  InputSameDT=on  OutDataTypeStr=Inherit: Inherit via internal rule
  Product : Product
  Product1 : Product
  Scope{,1..3} (4 alike) : Scope
  Stop Simulation : Stop
  camber : Outport
  wires:
  Fn/1 -> Product/1
  Product/1 -> Scope3/1, Product1/1
  n/1 -> Dot Product/1
  e0/1 -> Dot Product/2
  eLat/1 -> Product1/2
  Product1/1 -> Scope1/1, camber/1
  Dot Product/1 -> Scope/1, Scope2/1, Product/2, Compare To Constant/1  "sin_gamma"
  Compare To Constant/1 -> Stop Simulation/1

== system ThreeWheeledVehicle/Tire model/Force and moments block ==
  F_long : Inport
  F_lat : Inport  Port=2
  FnDisk : Inport  Port=3
  r : Inport  Port=4
  R : Inport  Port=5
  camber : Inport  Port=6
  phi_t : Inport  Port=7
  Add : Sum  Inputs=4
  Add1 : Sum
  Cross Product : vrlib/Utilities/Cross Product
      settings: SourceProductBaseCode=VR
  Demux : Demux  Outputs=3
  Demux1 : Demux  Outputs=3
  Product : Product  Inputs=/*  Multiplication=Matrix(*)
  Product1 : Product  Inputs=/*  Multiplication=Matrix(*)
  Scope : Scope  NumInputPorts=3
  Scope1 : Scope  NumInputPorts=3
  F : Outport
  M : Outport  Port=2
  wires:
  Add/1 -> Cross Product/2, Product/2
  R/1 -> Product1/1, Product/1
  Demux/3 -> Scope/3  "Mz"
  Demux/2 -> Scope/2  "My"
  Demux/1 -> Scope/1  "Mx"
  Cross Product/1 -> Add1/1
  camber/1 -> Add/4
  Product/1 -> Demux1/1, F/1
  Demux1/3 -> Scope1/3  "Fz"
  Demux1/2 -> Scope1/2  "Fy"
  Demux1/1 -> Scope1/1  "Fx"
  FnDisk/1 -> Add/1
  F_long/1 -> Add/2
  F_lat/1 -> Add/3
  Add1/1 -> Product1/2
  Product1/1 -> M/1, Demux/1
  r/1 -> Cross Product/1
  phi_t/1 -> Add1/2

== system ThreeWheeledVehicle/Tire model/Lateral Force A ==
  v_cx : Inport
  alpha : Inport  Port=2
  eLat : Inport  Port=3
  Constant : Constant  Value=sigma
  Constant1 : Constant  Value=sigma
  Gain : Gain  Gain=-C_F_alpha
  Integrator : Integrator
  Product{,1..4} (5 alike) : Product
  Scope : Scope
  Scope1 : Scope
  Sum : Sum  Inputs=|+-
  v_cx1 : InportShadow
  Fz : Outport
  wires:
  alpha/1 -> Scope1/1, Product/1  "input"
  v_cx/1 -> Product1/1
  Product/1 -> Sum/1
  Product1/1 -> Product/2
  Constant/1 -> Product1/2
  Sum/1 -> Integrator/1
  Integrator/1 -> Gain/1, Product2/1  "output"
  v_cx1/1 -> Product3/1
  Constant1/1 -> Product3/2
  Product3/1 -> Product2/2
  Product2/1 -> Sum/2
  Gain/1 -> Product4/1
  eLat/1 -> Product4/2
  Product4/1 -> Scope/1, Fz/1

== system ThreeWheeledVehicle/Tire model/Lateral slip with relaxation ==
  v_s : Inport
  eLat : Inport  Port=2
  v_cx : Inport  Port=3
  eLong : Inport  Port=4
  Dot Product : DotProduct  InputSameDT=on  OutDataTypeStr=Inherit: Inherit via internal rule
  Gain : Gain  Gain=1/sigma
  Gain1 : Gain  Gain=-C_F_alpha
  Integrator : Integrator
  Product : Product
  Product1 : Product
  Scope : Scope
  Scope1 : Scope
  Scope2 : Scope
  Sum : Sum  Inputs=|+-
  F_Lat : Outport
  wires:
  v_s/1 -> Dot Product/1
  eLat/1 -> Product1/2, Dot Product/2
  Dot Product/1 -> Scope1/1, Sum/1  "s2"
  Product/1 -> Sum/2
  Sum/1 -> Gain/1
  Gain/1 -> Integrator/1
  Integrator/1 -> Scope2/1, Gain1/1, Product/2  "alpha_F"
  Gain1/1 -> Product1/1
  Product1/1 -> Scope/1, F_Lat/1
  v_cx/1 -> Product/1

== system ThreeWheeledVehicle/Tire model/Longitudinal Force A ==
  v_cx : Inport
  kappa : Inport  Port=2
  eLong : Inport  Port=3
  Constant : Constant  Value=sigma
  Constant1 : Constant  Value=sigma
  Gain : Gain  Gain=-C_F_kappa
  Integrator : Integrator
  Product{,1..4} (5 alike) : Product
  Scope : Scope
  Scope1 : Scope
  Sum : Sum  Inputs=|+-
  v_cx1 : InportShadow
  Fx : Outport
  wires:
  kappa/1 -> Scope1/1, Product/1  "input"
  v_cx/1 -> Product1/1
  Product/1 -> Sum/1
  Product1/1 -> Product/2
  Constant/1 -> Product1/2
  Sum/1 -> Integrator/1
  Integrator/1 -> Gain/1, Product2/1  "output"
  v_cx1/1 -> Product3/1
  Constant1/1 -> Product3/2
  Product3/1 -> Product2/2
  Product2/1 -> Sum/2
  Gain/1 -> Product4/1
  eLong/1 -> Product4/2
  Product4/1 -> Scope/1, Fx/1

== system ThreeWheeledVehicle/Tire model/Longitudinal slip with relaxation ==
  v_s : Inport
  eLong : Inport  Port=2
  v_cx : Inport  Port=3
  Dot Product : DotProduct  InputSameDT=on  OutDataTypeStr=Inherit: Inherit via internal rule
  Gain : Gain  Gain=1/sigma
  Gain1 : Gain  Gain=-C_F_kappa
  Integrator : Integrator
  Product : Product
  Product1 : Product
  Scope : Scope
  Scope1 : Scope
  Sum : Sum  Inputs=|+-
  F_Long : Outport
  wires:
  v_s/1 -> Dot Product/1
  eLong/1 -> Product1/2, Dot Product/2
  Dot Product/1 -> Scope1/1, Sum/1  "s1"
  Product/1 -> Sum/2
  Sum/1 -> Gain/1
  Gain/1 -> Integrator/1
  Integrator/1 -> Gain1/1, Product/2  "kappa_F"
  Gain1/1 -> Product1/1
  Product1/1 -> Scope/1, F_Long/1
  v_cx/1 -> Product/1

== system ThreeWheeledVehicle/Tire model/Sensing ==
  PS-Simulink Converter{,1..9} (10 alike) : nesl_utility/PS-Simulink Converter  PhysicalDomain=network_engine_domain  SubClassName=ps_output  LeftPortType=input  RightPortType=output  PseudoPeriodic=off  Frequencies=[]  Unit=1  AffineConversion=off
  Scope : Scope
  Transform Sensor : sm_lib/Frames and Transforms/Transform Sensor  MeasurementFrame=Base  SenseAngle=off  SenseAxis=off  SenseAngle1=off  SenseAngle2=off  SenseAngle3=off  SenseQ=off  SenseR=on  SenseOmegaX=on  SenseOmegaY=on  SenseOmegaZ=on  SenseOmega1=off  SenseOmega2=off  SenseOmega3=off  SenseQDot=off  SenseRDot=off  SenseAlphaX=off  SenseAlphaY=off  SenseAlphaZ=off  SenseAlpha1=off  SenseAlpha2=off  SenseAlpha3=off  SenseQDDot=off  SenseRDDot=off  SenseX=on  SenseY=on  SenseZ=on  SenseRad=off  SenseAzim=off  SenseDist=off  SenseInc=off  SenseXDot=on  SenseYDot=on  SenseZDot=on  SenseRadDot=off  SenseAzimDot=off  SenseDistDot=off  SenseIncDot=off  SenseXDDot=off  SenseYDDot=off  SenseZDDot=off  SenseRadDDot=off  SenseAzimDDot=off  SenseDistDDot=off  SenseIncDDot=off
  Wheel : PMIOPort  Port=1  Side=Left
  Plane : PMIOPort  Port=2  Side=Left
  R : Outport
  x : Outport  Port=2
  y : Outport  Port=3
  z : Outport  Port=4
  vx : Outport  Port=5
  vy : Outport  Port=6
  vz : Outport  Port=7
  wx : Outport  Port=8
  wy : Outport  Port=9
  wz : Outport  Port=10
  wires:
  PS-Simulink Converter2/1 -> wy/1
  PS-Simulink Converter8/1 -> vy/1
  PS-Simulink Converter9/1 -> vz/1
  PS-Simulink Converter1/1 -> wx/1
  PS-Simulink Converter4/1 -> x/1
  PS-Simulink Converter7/1 -> vx/1
  PS-Simulink Converter3/1 -> wz/1
  PS-Simulink Converter5/1 -> y/1
  PS-Simulink Converter6/1 -> Scope/1, z/1
  PS-Simulink Converter/1 -> R/1
  connections:
  PS-Simulink Converter1/LConn1 -- Transform Sensor/RConn3
  PS-Simulink Converter4/LConn1 -- Transform Sensor/RConn6
  PS-Simulink Converter3/LConn1 -- Transform Sensor/RConn5
  PS-Simulink Converter9/LConn1 -- Transform Sensor/RConn11
  PS-Simulink Converter2/LConn1 -- Transform Sensor/RConn4
  PS-Simulink Converter6/LConn1 -- Transform Sensor/RConn8
  PS-Simulink Converter/LConn1 -- Transform Sensor/RConn2
  Transform Sensor/LConn1 -- Plane/RConn1
  Transform Sensor/RConn1 -- Wheel/RConn1
  PS-Simulink Converter5/LConn1 -- Transform Sensor/RConn7
  PS-Simulink Converter7/LConn1 -- Transform Sensor/RConn9
  PS-Simulink Converter8/LConn1 -- Transform Sensor/RConn10

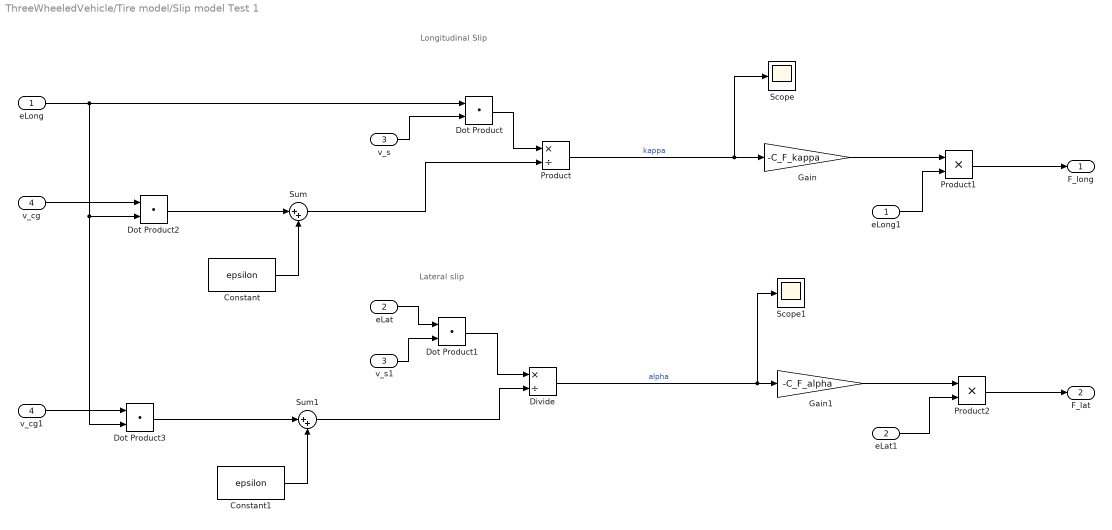
== system ThreeWheeledVehicle/Tire model/Slip model Test 1 ==
  note: Lateral slip
  note: Longitudinal Slip
  eLong : Inport
  eLat : Inport  Port=2
  v_s : Inport  Port=3
  v_cg : Inport  Port=4
  Constant : Constant  Value=epsilon
  Constant1 : Constant  Value=epsilon
  Divide : Product  Inputs=*/
  Dot Product{,1..3} (4 alike) : DotProduct  InputSameDT=on  OutDataTypeStr=Inherit: Inherit via internal rule
  Gain : Gain  Gain=-C_F_kappa
  Gain1 : Gain  Gain=-C_F_alpha
  Product : Product  Inputs=*/
  Product1 : Product
  Product2 : Product
  Scope : Scope
  Scope1 : Scope
  Sum : Sum  Inputs=|++
  Sum1 : Sum  Inputs=|++
  eLat1 : InportShadow  Port=2
  eLong1 : InportShadow
  v_cg1 : InportShadow  Port=4
  v_s1 : InportShadow  Port=3
  F_long : Outport
  F_lat : Outport  Port=2
  wires:
  eLong/1 -> Dot Product3/2, Dot Product2/2, Dot Product/1
  v_s/1 -> Dot Product/2
  Dot Product/1 -> Product/1
  Product/1 -> Scope/1, Gain/1  "kappa"
  eLat/1 -> Dot Product1/1
  v_s1/1 -> Dot Product1/2
  Dot Product1/1 -> Divide/1
  Divide/1 -> Scope1/1, Gain1/1  "alpha"
  Gain/1 -> Product1/1
  eLong1/1 -> Product1/2
  Gain1/1 -> Product2/1
  eLat1/1 -> Product2/2
  Product1/1 -> F_long/1
  Product2/1 -> F_lat/1
  Constant/1 -> Sum/2
  Sum/1 -> Product/2
  Constant1/1 -> Sum1/2
  Sum1/1 -> Divide/2
  v_cg/1 -> Dot Product2/1
  Dot Product2/1 -> Sum/1
  v_cg1/1 -> Dot Product3/1
  Dot Product3/1 -> Sum1/1

== system ThreeWheeledVehicle/Tire model/Slip model Test 2 ==
  note: Lateral slip
  note: Longitudinal Slip
  eLong : Inport
  eLat : Inport  Port=2
  v_s : Inport  Port=3
  v_cx : Inport  Port=4
  Divide : Product  Inputs=*/
  Dot Product : DotProduct  InputSameDT=on  OutDataTypeStr=Inherit: Inherit via internal rule
  Dot Product1 : DotProduct  InputSameDT=on  OutDataTypeStr=Inherit: Inherit via internal rule
  Gain : Gain  Gain=-C_F_kappa
  Gain1 : Gain  Gain=-C_F_alpha
  Product : Product  Inputs=*/
  Product1 : Product
  Product2 : Product
  Scope : Scope
  Scope1 : Scope
  eLat1 : InportShadow  Port=2
  eLong1 : InportShadow
  v_cx1 : InportShadow  Port=4
  v_s1 : InportShadow  Port=3
  F_long : Outport
  F_lat : Outport  Port=2
  kappa : Outport  Port=3
  alpha : Outport  Port=4
  wires:
  eLong/1 -> Dot Product/1
  Dot Product/1 -> Product/1
  eLat/1 -> Dot Product1/1
  Dot Product1/1 -> Divide/1
  Divide/1 -> alpha/1, Scope1/1, Gain1/1  "alpha"
  Gain/1 -> Product1/1
  eLong1/1 -> Product1/2
  Gain1/1 -> Product2/1
  eLat1/1 -> Product2/2
  Product1/1 -> F_long/1
  Product2/1 -> F_lat/1
  v_s/1 -> Dot Product/2
  v_s1/1 -> Dot Product1/2
  Product/1 -> Scope/1, kappa/1, Gain/1  "kappa"
  v_cx/1 -> Divide/2, Product/2

== system ThreeWheeledVehicle/Tire model/Slip velocity ==
  omega : Inport
  v_cg : Inport  Port=2
  r : Inport  Port=3
  Add : Sum
  Cross Product : vrlib/Utilities/Cross Product
      settings: SourceProductBaseCode=VR
  Scope : Scope
  Scope1 : Scope
  Scope4 : Scope
  v_s : Outport
  wires:
  omega/1 -> Cross Product/1
  Cross Product/1 -> Scope/1, Add/2  "v_r"
  r/1 -> Cross Product/2
  Add/1 -> Scope4/1, v_s/1
  v_cg/1 -> Scope1/1, Add/1  "V_x"

== system ThreeWheeledVehicle/Tire model/Turn Slip ==
  omega : Inport
  n : Inport  Port=2
  v_cx : Inport  Port=3
  Dot Product : DotProduct  InputSameDT=on  OutDataTypeStr=Inherit: Inherit via internal rule
  Gain : Gain  Gain=1/sigma
  Gain1 : Gain  Gain=-CM_phi
  Integrator : Integrator
  Product : Product
  Product1 : Product
  Sum : Sum  Inputs=|+-
  phi_t : Outport
  wires:
  omega/1 -> Dot Product/1
  n/1 -> Product/2, Dot Product/2
  Dot Product/1 -> Sum/1
  Sum/1 -> Gain/1
  Gain/1 -> Integrator/1
  Integrator/1 -> Product1/2, Gain1/1
  Gain1/1 -> Product/1
  Product/1 -> phi_t/1
  v_cx/1 -> Product1/1
  Product1/1 -> Sum/2

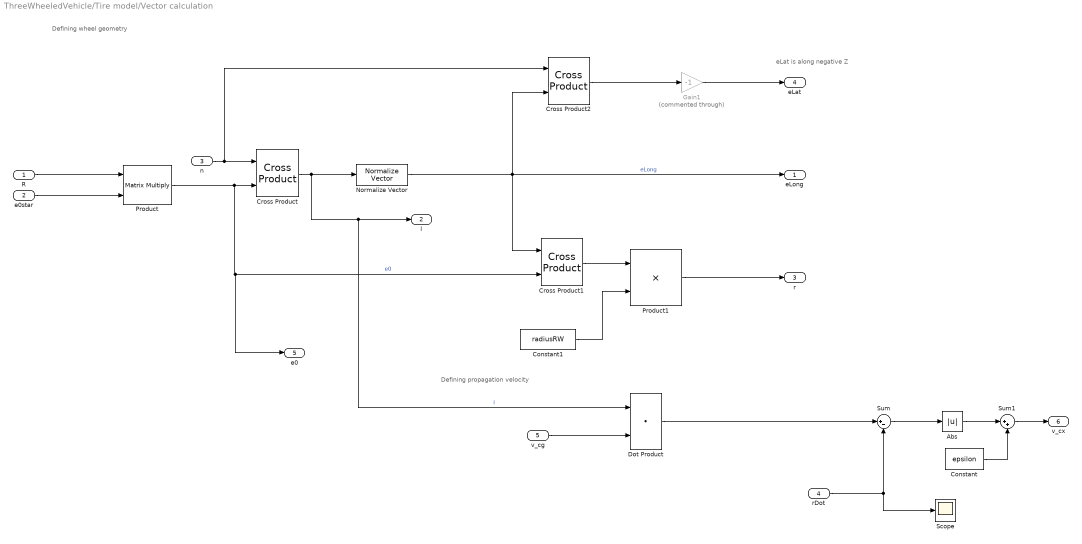
== system ThreeWheeledVehicle/Tire model/Vector calculation ==
  note: Defining propagation velocity
  note: Defining wheel geometry
  note: eLat is along
      | negative Z
  R : Inport
  e0star : Inport  Port=2
  n : Inport  Port=3
  rDot : Inport  Port=4
  v_cg : Inport  Port=5
  Abs : Abs  ZeroCross=off
  Constant : Constant  Value=epsilon
  Constant1 : Constant  Value=radiusRW
  Cross Product : vrlib/Utilities/Cross Product
      settings: SourceProductBaseCode=VR
  Cross Product1 : vrlib/Utilities/Cross Product
      settings: SourceProductBaseCode=VR
  Cross Product2 : vrlib/Utilities/Cross Product
      settings: SourceProductBaseCode=VR
  Dot Product : DotProduct  InputSameDT=on  OutDataTypeStr=Inherit: Inherit via internal rule
  Gain1 : Gain  Commented=through  Gain=-1
  Normalize Vector : vrlib/Utilities/Normalize Vector  maxzero=0
      settings: SourceProductName=Simulink 3D Animation  SourceProductBaseCode=VR
  Product : Product  Multiplication=Matrix(*)
  Product1 : Product
  Scope : Scope
  Sum : Sum  Inputs=|+-
  Sum1 : Sum  Inputs=|++
  eLong : Outport
  l : Outport  Port=2
  r : Outport  Port=3
  eLat : Outport  Port=4
  e0 : Outport  Port=5
  v_cx : Outport  Port=6
  wires:
  R/1 -> Product/1
  e0star/1 -> Product/2
  Product/1 -> Cross Product1/2, e0/1, Cross Product/2  "e0"
  n/1 -> Cross Product2/1, Cross Product/1
  Cross Product/1 -> Dot Product/1, l/1, Normalize Vector/1  "l"
  Normalize Vector/1 -> eLong/1, Cross Product2/2, Cross Product1/1  "eLong"
  Cross Product1/1 -> Product1/1
  Cross Product2/1 -> Gain1/1
  v_cg/1 -> Dot Product/2
  Dot Product/1 -> Sum/1
  Sum/1 -> Abs/1
  Abs/1 -> Sum1/1
  Sum1/1 -> v_cx/1
  Constant/1 -> Sum1/2
  Product1/1 -> r/1
  Gain1/1 -> eLat/1
  Constant1/1 -> Product1/2
  rDot/1 -> Sum/2, Scope/1

== system ThreeWheeledVehicle/Tire model/Verticle force ==
  note: Linear force law
  x_cg : Inport
  v_cg : Inport  Port=2
  r : Inport  Port=3
  n : Inport  Port=4
  Dot Product : DotProduct  InputSameDT=on  OutDataTypeStr=Inherit: Inherit via internal rule
  Dot Product1 : DotProduct  InputSameDT=on  OutDataTypeStr=Inherit: Inherit via internal rule
  Gain : Gain  Gain=-k_contact_RW
  Gain1 : Gain  Gain=-b_contact_RW
  Gain2 : Gain  Commented=through  Gain=-1
  Initial position of CP from ground : Constant  Value=[0 0 0]'
  Product : Product
  Scope : Scope
  Sum : Sum  Inputs=|++
  Sum1 : Sum  Inputs=|+-
  Sum2 : Sum
  Fn : Outport
  FnDisk : Outport  Port=2
  wires:
  x_cg/1 -> Sum/1
  Sum/1 -> Scope/1, Sum1/1  "CP position from ground"
  Initial position of CP from ground/1 -> Sum1/2
  Sum1/1 -> Dot Product/1
  Dot Product/1 -> Gain/1  "pen"
  v_cg/1 -> Dot Product1/2
  Dot Product1/1 -> Gain1/1  "pentration velocity"
  Gain1/1 -> Sum2/2
  Sum2/1 -> Fn/1, Gain2/1
  n/1 -> Product/2, Dot Product1/1, Dot Product/2
  Gain/1 -> Sum2/1
  r/1 -> Sum/2
  Product/1 -> FnDisk/1
  Gain2/1 -> Product/1

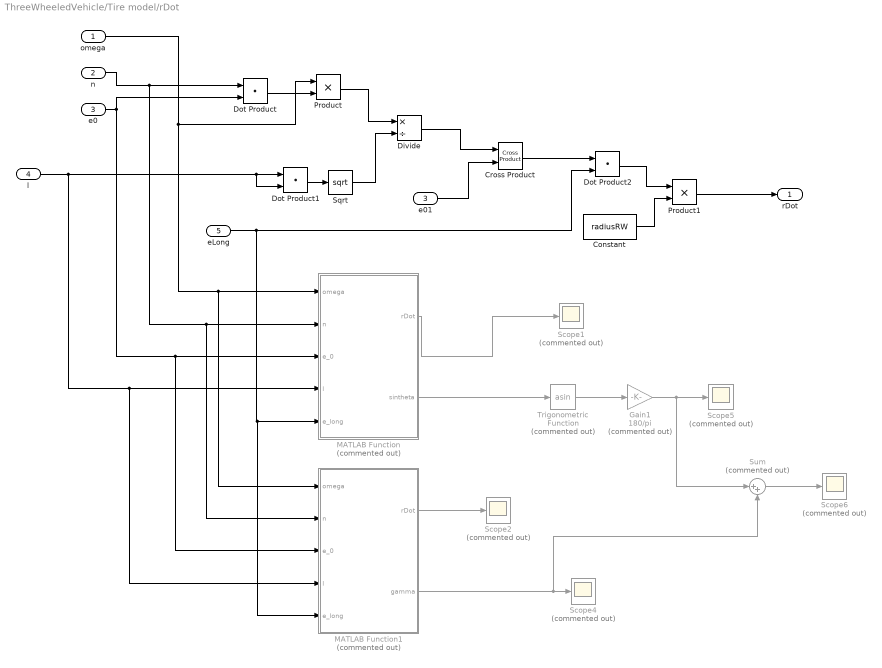
== system ThreeWheeledVehicle/Tire model/rDot ==
  omega : Inport
  n : Inport  Port=2
  e0 : Inport  Port=3
  l : Inport  Port=4
  eLong : Inport  Port=5
  Constant : Constant  Value=radiusRW
  Cross Product : vrlib/Utilities/Cross Product
      settings: SourceProductBaseCode=VR
  Divide : Product  Inputs=*/
  Dot Product : DotProduct  InputSameDT=on  OutDataTypeStr=Inherit: Inherit via internal rule
  Dot Product1 : DotProduct  InputSameDT=on  OutDataTypeStr=Inherit: Inherit via internal rule
  Dot Product2 : DotProduct  InputSameDT=on  OutDataTypeStr=Inherit: Inherit via internal rule
  Gain1 : Gain  Commented=on  Gain=180/pi
  MATLAB Function : MATLAB Function  Commented=on  TreatAsAtomicUnit=on
  MATLAB Function1 : MATLAB Function  Commented=on  TreatAsAtomicUnit=on
  Product : Product
  Product1 : Product
  Scope{1..2,4..6} (5 alike) : Scope  Commented=on
  Sqrt : Sqrt  SaturateOnIntegerOverflow=on
  Sum : Sum  Commented=on  Inputs=|++
  Trigonometric Function : Trigonometry  Commented=on  Operator=asin
  e01 : InportShadow  Port=3
  rDot : Outport
  wires:
  n/1 -> MATLAB Function1/2(n), MATLAB Function/2(n), Dot Product/1
  e0/1 -> MATLAB Function1/3(e_0), MATLAB Function/3(e_0), Dot Product/2
  Dot Product/1 -> Product/2
  omega/1 -> MATLAB Function1/1(omega), MATLAB Function/1(omega), Product/1
  Product/1 -> Divide/1
  l/1 -> MATLAB Function1/4(l), MATLAB Function/4(l), Dot Product1/2, Dot Product1/1
  Dot Product1/1 -> Sqrt/1
  Sqrt/1 -> Divide/2
  Divide/1 -> Cross Product/1
  e01/1 -> Cross Product/2
  Cross Product/1 -> Dot Product2/1
  eLong/1 -> MATLAB Function1/5(e_long), MATLAB Function/5(e_long), Dot Product2/2
  Dot Product2/1 -> Product1/1
  Constant/1 -> Product1/2
  MATLAB Function/1(rDot) -> Scope1/1
  MATLAB Function1/1(rDot) -> Scope2/1
  Product1/1 -> rDot/1
  MATLAB Function1/2(gamma) -> Sum/2, Scope4/1
  MATLAB Function/2(sintheta) -> Trigonometric Function/1
  Trigonometric Function/1 -> Gain1/1
  Gain1/1 -> Sum/1, Scope5/1
  Sum/1 -> Scope6/1

== system ThreeWheeledVehicle/Tire model1/Camber thrust ==
  Fn : Inport
  eLat : Inport  Port=2
  n : Inport  Port=3
  e0 : Inport  Port=4
  Compare To Constant : simulink/Logic and Bit Operations/Compare To Constant  relop=<=  const=-1  OutDataTypeStr=boolean
  Dot Product : DotProduct  InputSameDT=on  OutDataTypeStr=Inherit: Inherit via internal rule
  Product : Product
  Product1 : Product
  Scope : Scope
  Scope1 : Scope
  Scope3 : Scope
  Stop Simulation : Stop
  camber : Outport
  wires:
  Fn/1 -> Product/1
  Product/1 -> Scope3/1, Product1/1
  n/1 -> Dot Product/1
  e0/1 -> Dot Product/2
  eLat/1 -> Product1/2
  Product1/1 -> Scope1/1, camber/1
  Dot Product/1 -> Scope/1, Product/2, Compare To Constant/1  "sin_gamma"
  Compare To Constant/1 -> Stop Simulation/1

== system ThreeWheeledVehicle/Tire model1/Force and moments block ==
  F_long : Inport
  F_lat : Inport  Port=2
  FnDisk : Inport  Port=3
  r : Inport  Port=4
  R : Inport  Port=5
  camber : Inport  Port=6
  phi_t : Inport  Port=7
  Add : Sum  Inputs=4
  Add1 : Sum
  Cross Product : vrlib/Utilities/Cross Product
      settings: SourceProductBaseCode=VR
  Demux : Demux  Outputs=3
  Demux1 : Demux  Outputs=3
  Product : Product  Inputs=/*  Multiplication=Matrix(*)
  Product1 : Product  Inputs=/*  Multiplication=Matrix(*)
  Scope : Scope  NumInputPorts=3
  Scope1 : Scope  NumInputPorts=3
  F : Outport
  M : Outport  Port=2
  wires:
  Add/1 -> Cross Product/2, Product/2
  R/1 -> Product1/1, Product/1
  Demux/3 -> Scope/3  "Mz"
  Demux/2 -> Scope/2  "My"
  Demux/1 -> Scope/1  "Mx"
  Cross Product/1 -> Add1/1
  camber/1 -> Add/4
  Product/1 -> Demux1/1, F/1
  Demux1/3 -> Scope1/3  "Fz"
  Demux1/2 -> Scope1/2  "Fy"
  Demux1/1 -> Scope1/1  "Fx"
  FnDisk/1 -> Add/1
  F_long/1 -> Add/2
  F_lat/1 -> Add/3
  Add1/1 -> Product1/2
  Product1/1 -> M/1, Demux/1
  r/1 -> Cross Product/1
  phi_t/1 -> Add1/2
